simulink model "ChargePump5"  (R2024a)
settings: Solver=ode23t  StartTime=0.0  StopTime=0.5  RelTol=1e-3
libraries: fl_lib x10, nesl_utility x6, ee_lib x2
settings Model: Creator=CHangLeo  LastModifiedBy=CHangLeo

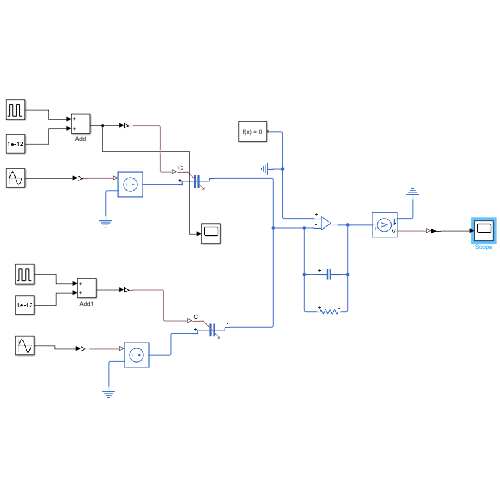
[thumbnail: Simulink's stored preview of the top-level diagram]
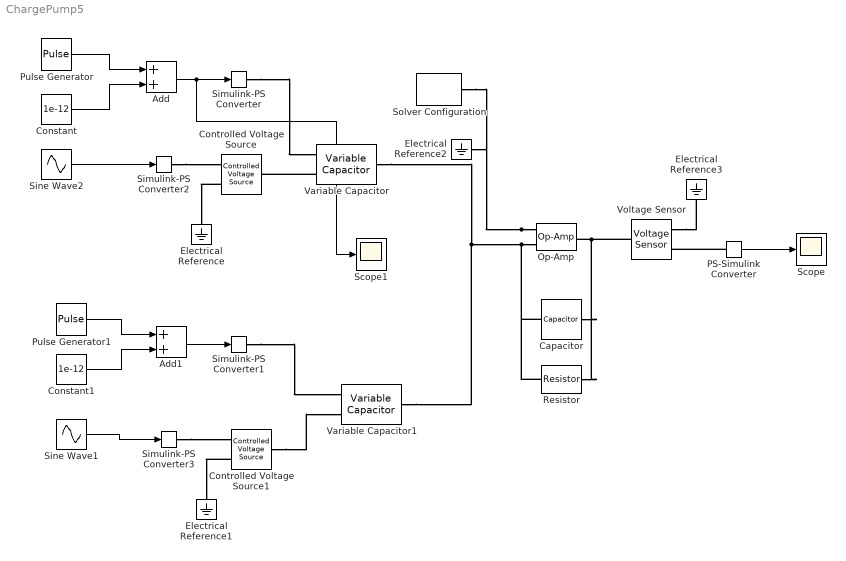
== system ChargePump5 ==
  Add : Sum
  Add1 : Sum
  Capacitor : fl_lib/Electrical/Electrical Elements/Capacitor  c=10000 pF  r=1e-6 Ohm  g=0 1/Ohm  i_specify=off  i_priority=None  i=0 A  i_nominal_specify=off  i_nominal_value=1  i_nominal_unit=A  v_specify=off  v_priority=None  v=0 V  v_nominal_specify=off  v_nominal_value=1  v_nominal_unit=V  vc_specify=off  vc_priority=High  vc=0 V  vc_nominal_specify=off  vc_nominal_value=1  vc_nominal_unit=V
  Constant : Constant  Value=1e-12
  Constant1 : Constant  Value=1e-12
  Controlled Voltage Source : fl_lib/Electrical/Electrical Sources/Controlled Voltage Source
  Controlled Voltage Source1 : fl_lib/Electrical/Electrical Sources/Controlled Voltage Source
  Electrical Reference{,1..3} (4 alike) : fl_lib/Electrical/Electrical Elements/Electrical Reference
  Op-Amp : fl_lib/Electrical/Electrical Elements/Op-Amp  outI_specify=off  outI_priority=None  outI=0 A  outI_nominal_specify=off  outI_nominal_value=1  outI_nominal_unit=A
  PS-Simulink Converter : nesl_utility/PS-Simulink Converter  PhysicalDomain=network_engine_domain  SubClassName=ps_output  LeftPortType=input  RightPortType=output  PseudoPeriodic=off  Frequencies=[]  VectorFormat=1-D array  Unit=inherit  AffineConversion=off
  Pulse Generator : DiscretePulseGenerator  PulseType=Time based  Amplitude=1e-15  Period=0.2  PulseWidth=50
  Pulse Generator1 : DiscretePulseGenerator  PulseType=Time based  Amplitude=-1e-15  Period=0.2  PulseWidth=50
  Resistor : fl_lib/Electrical/Electrical Elements/Resistor  R=100 MOhm  i_specify=off  i_priority=None  i=0 A  i_nominal_specify=off  i_nominal_value=1  i_nominal_unit=A  v_specify=off  v_priority=None  v=0 V  v_nominal_specify=off  v_nominal_value=1  v_nominal_unit=V
  Scope : Scope
  Scope1 : Scope
  Simulink-PS Converter{,1..3} (4 alike) : nesl_utility/Simulink-PS Converter  PhysicalDomain=network_engine_domain  SubClassName=ps_input  LeftPortType=input  RightPortType=output  PseudoPeriodic=off  Frequencies=[]  NoiseDistribution=none  NoiseParameters=[]  Unit=1  AffineConversion=off  FilteringAndDerivatives=provide  SimscapeFilterOrder=1  InputFilterTimeConstant=0.001  UdotUserProvided=0
  Sine Wave1 : Sin  Frequency=1000  Phase=pi  SampleTime=0
  Sine Wave2 : Sin  Frequency=1000  SampleTime=0
  Solver Configuration : nesl_utility/Solver Configuration  PhysicalDomain=network_engine_domain  SubClassName=solver  LeftPortType=input  RightPortType=generic  Tones=[]  Harmonics=[]  SimulateNoise=off  Profile=off  UseLocalSampling=off  EnableSwitchedLinearOptims=on  FrequencyDomain=off  UseCCode=off  RelTol=0.001  AbsTol=1e-06  MinStep=1e-09  ToWorkspace=off  RevertToSquareIcSolve=off  NumHomotopyIterations=100  PhasorMode=off  PhasorModeNumHarmonics=1  ConsistencySolver=NEWTON_FTOL  IndexReductionMethod=DerivativeReplacement  DoDC=off  ResidualTolerance=1e-09  ConsistencyTolSource=GLOBAL  ConsistencyAbsTol=0.001  ConsistencyRelTol=0.001  ConsistencyTolFactor=0.001  UseLocalSolver=off  LocalSolverChoice=NE_BACKWARD_EULER_ADVANCER  ResolveIndetEquations=on  FunctionEvalNumThread=1  LocalSolverSampleTime=0.001  DoFixedCost=off  MaxNonlinIter=3  MaxModeIter=2  ComputeImpulses=off  ImpulseIterations=2  LinearAlgebra=auto  LinearAlgebraNumThread=0  EquationFormulation=NE_TIME_EF  DelaysMemoryBudget=1024  AutomaticFiltering=on  FilteringTimeConstant=0.001  PartitionStorageMethod=AS_NEEDED  PartitionMemoryBudget=1024  PartitionMethod=ROBUST  MultibodyUseLocalSolver=off  MultibodyLocalSolverChoice=ODE1  MultibodyLocalSolverSampleTime=0.001
  Variable Capacitor : ee_lib/Passive/Variable Capacitor  prm=1  Cmin=0.001 pF  r=1e-6 Ohm  v0=0 V  q0=0 C
      settings: InternalSimscapePortConfiguration="{\"Bottom\":[],\"Left\":[{\"id\":\"C\",\"label\":\"C\",\"type\":\"input\"},{\"id\":\"p\",\"label\":\"+\",\"type\":\"foundation.electrical.electrical\"}],\"Right\":[{\"id\":\"n\",\"label\":\"-\",\"type\":\"foundation.electrical.electrical\"}],\"Top\":[]}"
  Variable Capacitor1 : ee_lib/Passive/Variable Capacitor  prm=1  Cmin=0.001 pF  r=1e-6 Ohm  v0=0 V  q0=0 C
      settings: InternalSimscapePortConfiguration="{\"Bottom\":[],\"Left\":[{\"id\":\"C\",\"label\":\"C\",\"type\":\"input\"},{\"id\":\"p\",\"label\":\"+\",\"type\":\"foundation.electrical.electrical\"}],\"Right\":[{\"id\":\"n\",\"label\":\"-\",\"type\":\"foundation.electrical.electrical\"}],\"Top\":[]}"
  Voltage Sensor : fl_lib/Electrical/Electrical Sensors/Voltage Sensor
  wires:
  Pulse Generator/1 -> Add/1
  Constant/1 -> Add/2
  Pulse Generator1/1 -> Add1/1
  Constant1/1 -> Add1/2
  Add/1 -> Scope1/1, Simulink-PS Converter/1
  Add1/1 -> Simulink-PS Converter1/1
  Sine Wave2/1 -> Simulink-PS Converter2/1
  Sine Wave1/1 -> Simulink-PS Converter3/1
  PS-Simulink Converter/1 -> Scope/1
  connections:
  Simulink-PS Converter2/RConn1 -- Controlled Voltage Source/RConn1
  Simulink-PS Converter3/RConn1 -- Controlled Voltage Source1/RConn1
  Controlled Voltage Source/RConn2 -- Electrical Reference/LConn1
  Controlled Voltage Source1/RConn2 -- Electrical Reference1/LConn1
  Simulink-PS Converter1/RConn1 -- Variable Capacitor1/LConn1
  Controlled Voltage Source1/LConn1 -- Variable Capacitor1/LConn2
  Variable Capacitor1/RConn1 -- Variable Capacitor/RConn1 -- Resistor/LConn1 -- Capacitor/LConn1 -- Op-Amp/LConn2
  Op-Amp/LConn1 -- Solver Configuration/RConn1 -- Electrical Reference2/LConn1
  Voltage Sensor/LConn1 -- Resistor/RConn1 -- Capacitor/RConn1 -- Op-Amp/RConn1
  Voltage Sensor/RConn2 -- Electrical Reference3/LConn1
  PS-Simulink Converter/LConn1 -- Voltage Sensor/RConn1
  Variable Capacitor/LConn2 -- Controlled Voltage Source/LConn1
  Simulink-PS Converter/RConn1 -- Variable Capacitor/LConn1
